simulink model "slexSVMIonospherePredictExample"  (R2017a)
settings: Solver=FixedStepDiscrete  StartTime=0.0  StopTime=radarReturnInput.time(end)  FixedStep=1  RelTol=1e-3
PreLoadFcn:
  | load(fullfile(matlabroot,'help','toolbox','stats','examples','radarReturnInput.mat'))
settings Model: Creator=The MathWorks, Inc.  LastModifiedBy=Felipe
settings DataIOCC: ExternalInput=radarReturnInput  LoadExternalInput=on  SignalLoggingName=svmlogsout
settings OptimizationCC: DefaultParameterBehavior=Inlined  LifeSpan=inf
settings DebuggingCC: ParameterTunabilityLossMsg=error  SFExecutionAtInitializationDiag=none
settings SFSimCC: CompileTimeRecursionLimit=0  EnableRuntimeRecursion=off  MATLABDynamicMemAlloc=off
settings RTWCC: SystemTargetFile=ert.tlc  TemplateMakefile=ert_default_tmf  Description=Embedded Coder  GenerateReport=on  IncludeHyperlinkInReport=on  LaunchReport=on  GenerateTraceInfo=on  GenerateTraceReport=on  GenerateTraceReportSl=on  GenerateTraceReportSf=on  GenerateTraceReportEml=on
settings CodeAppCC: ForceParamTrailComments=on  IgnoreCustomStorageClasses=off  OperatorAnnotations=on  SimulinkDataObjDesc=on  SFDataObjDesc=on  MATLABFcnDesc=on  InsertBlockDesc=on  MATLABSourceComments=on
settings ERTTargetCC: TargetLangStandard=C99 (ISO)  MultiwordLength=2048  GenerateSampleERTMain=on  InlinedParameterPlacement=NonHierarchical  ERTCustomFileTemplate=example_file_process.tlc
settings ConfigComp: CovMetricSettings=dswe

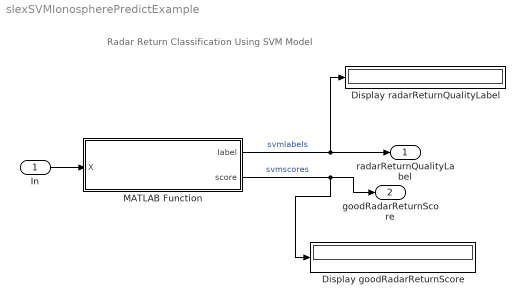
== system slexSVMIonospherePredictExample ==
  note: Radar Return Classification Using SVM Model
  In : Inport  PortDimensions=[34]
  Display goodRadarReturnScore : Display
  Display radarReturnQualityLabel : Display
  MATLAB Function : MATLAB Function  TreatAsAtomicUnit=on
  radarReturnQualityLabel : Outport
  goodRadarReturnScore : Outport  Port=2
  wires:
  In/1 -> MATLAB Function/1(X)
  MATLAB Function/1(label) -> radarReturnQualityLabel/1, Display radarReturnQualityLabel/1  "svmlabels"
  MATLAB Function/2(score) -> goodRadarReturnScore/1, Display goodRadarReturnScore/1  "svmscores"

== matlab function slexSVMIonospherePredictExample/MATLAB Function ==
  data: label output; X input size=[1,34]; score output
function [label,score] = svmIonospherePredict(X) %#codegen
%svmIonospherePredict Predict radar-return quality using SVM model
%   svmIonospherePredict predicts labels and estimates classification
%   scores of the radar returns in the numeric matrix of preditor data X
%   using the compact SVM model in the file SVMIonosphere.mat.  Rows of X
%   correspond to observations and columns to predictor variables.  label
%   is the predicted label and score is the confidence measure for
%   classifying the radar-return quality as good.
%
% Copyright 2016 The MathWorks Inc.
Mdl = loadCompactModel('SVMIonosphere');
[label,bothscores] = predict(Mdl,X);
score = bothscores(:,2);
end
